simulink model "test"  (R2020a)
settings: Solver=VariableStepAuto  StartTime=0.0  StopTime=1.0  RelTol=1e-3
model workspace (MAT data in the model file):
  PnFrequencyOffset_375 = [30000 100000 1000000 3000000 10000000]
libraries: simulink x1, dspadpt3 x1, dspsrcs4 x1
settings Model: Creator=a'su's  LastModifiedBy=a'su's
settings SolverCC: ZeroCrossAlgorithm=Adaptive
settings DebuggingCC: IgnoredZcDiagnostic=none

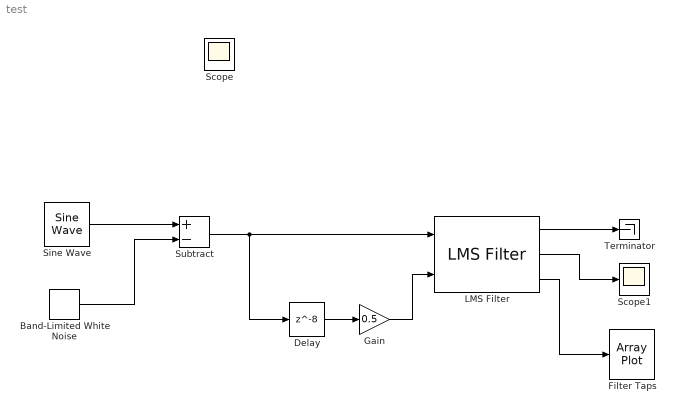
== system test ==
  Band-Limited White Noise : simulink/Sources/Band-Limited White Noise  Cov=0.5e-4  Ts=0.001  seed=[23341]
  Delay : Delay  DelayLength=8
  Filter Taps : ArrayPlot
  Gain : Gain  Gain=0.5
  LMS Filter : dspadpt3/LMS Filter  Algo=Normalized LMS  L=14  stepflag=Dialog  mu=0.3  leakage=1.0  ic=0  Adapt=off  resetflag=None  weights=on  addnparflag=off  roundingMode=Floor  overflowMode=off  secondCoeffMode=Binary point scaling  secondCoeffWordLength=2  secondCoeffFracLength=15  prodOutput2Mode=Binary point scaling  prodOutput2FracLength=20  prodOutput3Mode=Binary point scaling  prodOutput3FracLength=20  prodOutput4Mode=Binary point scaling  prodOutput4FracLength=20  quotientMode=Binary point scaling  quotientFracLength=20  accum2Mode=Binary point scaling  accum2FracLength=20
      settings: SourceProductBaseCode=DS
  Scope1 : Scope
  Sine Wave : dspsrcs4/Sine Wave  Amplitude=1  Frequency=50  Phase=0  SampleMode=Discrete  OutComplex=Real  CompMethod=Trigonometric fcn  TableSize=Speed  SampleTime=1e-5  SamplesPerFrame=1  ResetState=Restart at time zero  OutputFrames=off  dataType=double  wordLen=16  udDataType=sfix(16)  fracBitsMode=Best precision  numFracBits=15  OutDataTypeStr=double  LastOutDataTypeStr=double
  Subtract : Sum  Inputs=+-
  Terminator : Terminator
  Scope : Scope
  wires:
  Subtract/1 -> Delay/1, LMS Filter/1
  LMS Filter/1 -> Terminator/1
  Delay/1 -> Gain/1
  Gain/1 -> LMS Filter/2
  Sine Wave/1 -> Subtract/1
  Band-Limited White Noise/1 -> Subtract/2
  LMS Filter/2 -> Scope1/1
  LMS Filter/3 -> Filter Taps/1
